simulink model "Modelo_tarea2"  (R2024b)
settings: Solver=VariableStepAuto  StartTime=0.0  StopTime=20  RelTol=1e-3
undefined symbols (not defined in the file): a, alpha, beta_f, g_m, gamma, x1_0, x2_0, xr
settings Model: Creator=juanm  LastModifiedBy=juanm

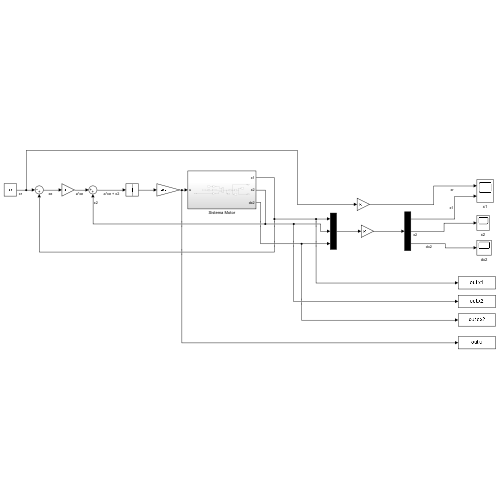
[thumbnail: Simulink's stored preview of the top-level diagram]
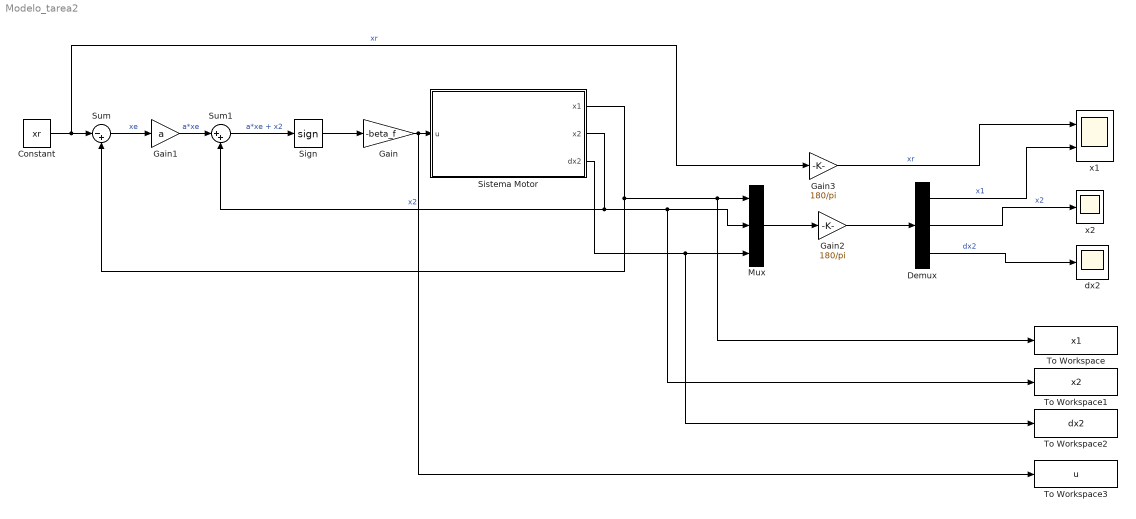
== system Modelo_tarea2 ==
  Constant : Constant  Value=xr
  Demux : Demux  Outputs=3
  Gain : Gain  Gain=-beta_f
  Gain1 : Gain  Gain=a
  Gain2 : Gain  Gain=180/pi
  Gain3 : Gain  Gain=180/pi
  Mux : Mux  Inputs=3
  Sign : Signum  ZeroCross=off
  Sistema Motor : Subsystem
  Sum : Sum  Inputs=|-+
  Sum1 : Sum  Inputs=|++
  To Workspace : ToWorkspace  VariableName=x1  SaveFormat=Timeseries  SampleTime=-1
  To Workspace1 : ToWorkspace  VariableName=x2  SaveFormat=Timeseries  SampleTime=-1
  To Workspace2 : ToWorkspace  VariableName=dx2  SaveFormat=Timeseries  SampleTime=-1
  To Workspace3 : ToWorkspace  VariableName=u  SaveFormat=Timeseries  SampleTime=-1
  dx2 : Scope
  x1 : Scope  NumInputPorts=2
  x2 : Scope
  wires:
  Gain/1 -> To Workspace3/1, Sistema Motor/1(u)
  Sistema Motor/1(x1) -> To Workspace/1, Mux/1, Sum/2
  Sum/1 -> Gain1/1  "xe"
  Sistema Motor/2(x2) -> To Workspace1/1, Mux/2, Sum1/2  "x2"
  Gain1/1 -> Sum1/1  "a*xe"
  Sum1/1 -> Sign/1  "a*xe + x2"
  Sign/1 -> Gain/1
  Gain2/1 -> Demux/1
  Mux/1 -> Gain2/1
  Sistema Motor/3(dx2) -> To Workspace2/1, Mux/3
  Demux/1 -> x1/2  "x1"
  Demux/2 -> x2/1  "x2"
  Demux/3 -> dx2/1  "dx2"
  Constant/1 -> Sum/1, Gain3/1  "xr"
  Gain3/1 -> x1/1  "xr"

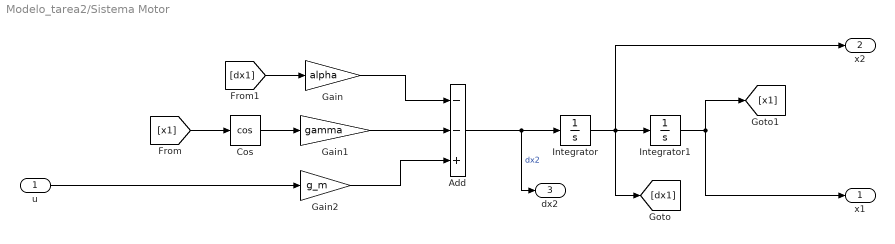
== system Modelo_tarea2/Sistema Motor ==
  u : Inport
  Add : Sum  Inputs=--+
  Cos : Trigonometry  Operator=cos
  Gain : Gain  Gain=alpha
  Gain1 : Gain  Gain=gamma
  Gain2 : Gain  Gain=g_m
  Integrator : Integrator  InitialCondition=x2_0
  Integrator1 : Integrator  InitialCondition=x1_0
  x1 : Outport
  x2 : Outport  Port=2
  dx2 : Outport  Port=3
  wires:
  Add/1 -> dx2/1, Integrator/1  "dx2"
  Gain1/1 -> Add/2
  Integrator1/1 -> x1/1, [x1]
  Gain2/1 -> Add/3
  Cos/1 -> Gain1/1
  Gain/1 -> Add/1
  Integrator/1 -> x2/1, [dx1], Integrator1/1
  u/1 -> Gain2/1
  [x1] -> Cos/1
  [dx1] -> Gain/1
